simulink model "model"  (R2018b)
settings: Solver=FixedStepAuto  StartTime=0.0  StopTime=sim_time  FixedStep=Ts/10  RelTol=1e-3
StopFcn:
  | %figure;plot(true_position.Data(:,1),true_position.Data(:,2))
values from neighbouring files (symbols this model uses):
  b = 1.115    [main.m]
  bike_params = [g h b a lambda m]    [main.m]
  chalmers = 1    [main.m]
  complementary = 0.985    [main.m]
  D_balancing = 0.0646    [main.m]
  D_heading = 0.01    [main.m]
  D_lateral = 0.01    [main.m]
  g = 9.82    [main.m]
  heading_control = 1    [main.m]
  I_balancing = 1.327    [main.m]
  I_heading = -0.01    [main.m]
  I_lateral = 0    [main.m]
  IMU_height = 0.2    [main.m]
  initial_roll = deg2rad(2)    [main.m]
  initial_rollrate = deg2rad(0)    [main.m]
  initial_steering = deg2rad(0)    [main.m]
  initial_x = 0    [main.m]
  initial_y = 0    [main.m]
  lambda = deg2rad(90-24)    [main.m]
  lateral_control = 0    [main.m]
  mdh = 0    [main.m]
  P_balancing = 3.418    [main.m]
  P_heading = -0.1    [main.m]
  P_lateral = -0.07    [main.m]
  path_tracking = 1    [main.m]
  roll_rate_coef = 0.9    [main.m]
  Ts = 0.01    [main.m]
  v = v_vec(i)    [bike_linear_analysis_balancing.m]    (also in main.m = 3.88888888889)
undefined symbols (not defined in the file or in its folder): A, B, b_compFilter, C, cumulative_dist_along_path, D, IMU_height_model, initial_states, lambda_compFilter, max_roll, min_roll, num_tf_steering, path_x, path_y, Ts_IMU
libraries: simulink x6, dspsigops x2
settings Model: Creator=maximef  LastModifiedBy=maximef

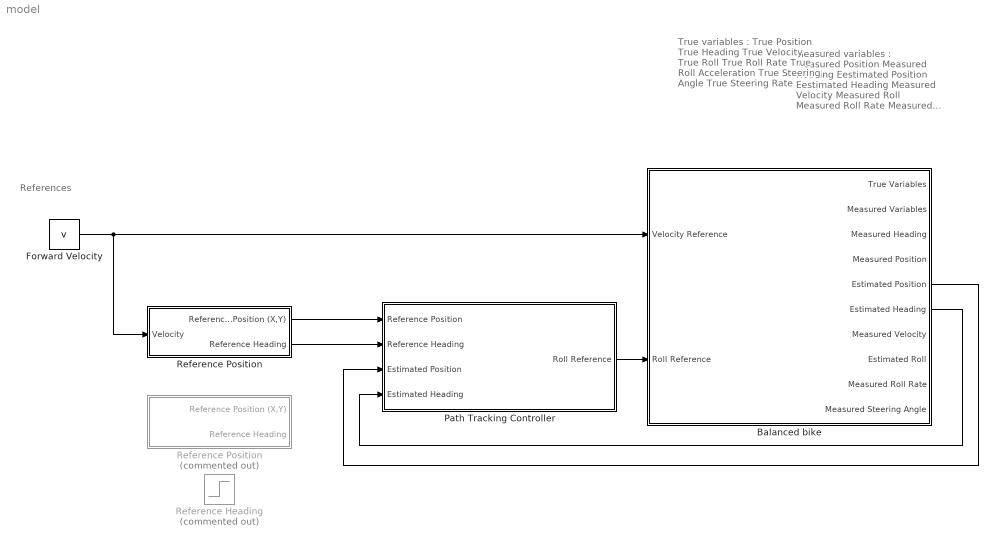
== system model ==
  note: References
  note: Measured variables :
      | Measured Position
      | Measured Heading
      | Eestimated Position
      | Eestimated Heading
      | Measured Velocity
      | Measured Roll
      | Measured Roll Rate
      | Measured Steering Angle
  note: True variables :
      | True Position
      | True Heading
      | True Velocity
      | True Roll
      | True Roll Rate
      | True Roll Acceleration
      | True Steering Angle
      | True Steering Rate
  Balanced bike : Subsystem
  Forward Velocity : Constant  Value=v
  Path Tracking Controller : Subsystem
  Reference Heading : Step  Commented=on  SampleTime=0
  Reference Position : Subsystem  Commented=on
  "Reference Position " : Subsystem
  wires:
  "Reference Position "/1(Reference Position (X,Y)) -> Path Tracking Controller/1(Reference Position)
  "Reference Position "/2(Reference Heading) -> Path Tracking Controller/2(Reference Heading)
  Forward Velocity/1 -> "Reference Position "/1(Velocity), Balanced bike/1(Velocity Reference)
  Path Tracking Controller/1(Roll Reference) -> Balanced bike/2(Roll Reference)
  Balanced bike/5(Estimated Position) -> Path Tracking Controller/3(Estimated Position)
  Balanced bike/6(Estimated Heading) -> Path Tracking Controller/4(Estimated Heading)

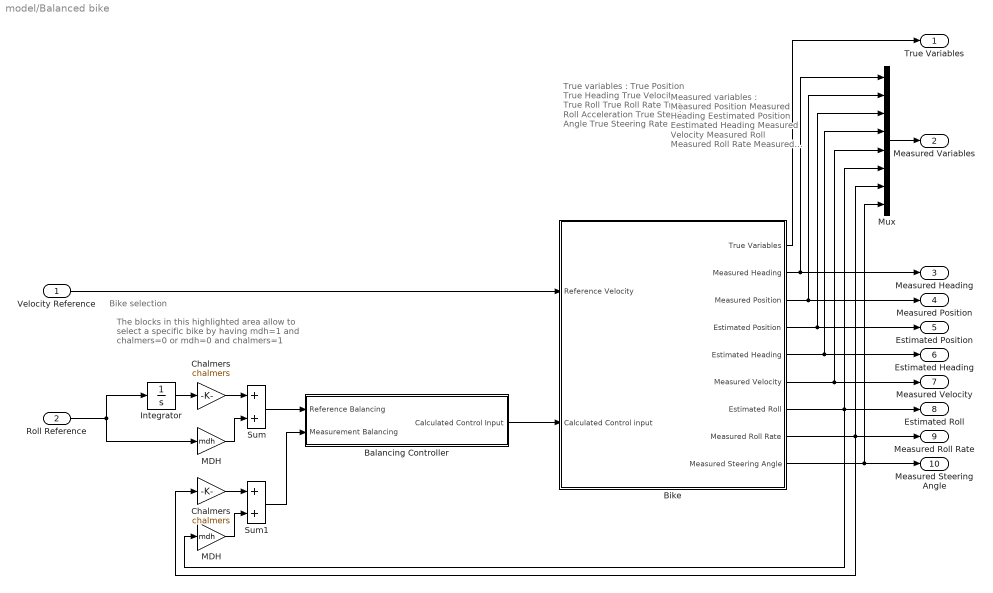
== system model/Balanced bike ==
  note: The blocks in this highlighted area allow
      | to select a specific bike by having
      | mdh=1 and chalmers=0
      | or
      | mdh=0 and chalmers=1
  note: Bike selection
  note: True variables :
      | True Position
      | True Heading
      | True Velocity
      | True Roll
      | True Roll Rate
      | True Roll Acceleration
      | True Steering Angle
      | True Steering Rate
  note: Measured variables :
      | Measured Position
      | Measured Heading
      | Eestimated Position
      | Eestimated Heading
      | Measured Velocity
      | Measured Roll
      | Measured Roll Rate
      | Measured Steering Angle
  Velocity Reference : Inport
  Roll Reference : Inport  Port=2
  Balancing Controller : Subsystem
  Bike : Subsystem
  Chalmers : Gain  Gain=chalmers
  "Chalmers " : Gain  Gain=chalmers
  Integrator : Integrator  InitialCondition=initial_roll
  MDH : Gain  Gain=mdh
  "MDH " : Gain  Gain=mdh
  Mux : Mux  Inputs=8
  Sum : Sum
  Sum1 : Sum
  True Variables : Outport
  Measured Variables : Outport  Port=2
  Measured Heading : Outport  Port=3
  Measured Position : Outport  Port=4
  Estimated Position : Outport  Port=5
  Estimated Heading : Outport  Port=6
  Measured Velocity : Outport  Port=7
  Estimated Roll : Outport  Port=8
  Measured Roll Rate : Outport  Port=9
  Measured Steering Angle : Outport  Port=10
  wires:
  Bike/4(Estimated Position) -> Mux/3, Estimated Position/1
  Bike/3(Measured Position) -> Measured Position/1, Mux/2
  Balancing Controller/1(Calculated Control Input) -> Bike/2(Calculated Control input)
  Velocity Reference/1 -> Bike/1(Reference Velocity)
  Bike/5(Estimated Heading) -> Mux/4, Estimated Heading/1
  Bike/2(Measured Heading) -> Mux/1, Measured Heading/1
  Roll Reference/1 -> Integrator/1, MDH/1
  Chalmers/1 -> Sum/1
  Sum1/1 -> Balancing Controller/2(Measurement Balancing)
  Bike/7(Estimated Roll) -> Mux/6, "MDH "/1, Estimated Roll/1
  Integrator/1 -> Chalmers/1
  Bike/6(Measured Velocity) -> Mux/5, Measured Velocity/1
  Bike/8(Measured Roll Rate) -> Mux/7, "Chalmers "/1, Measured Roll Rate/1
  Bike/9(Measured Steering Angle) -> Mux/8, Measured Steering Angle/1
  "Chalmers "/1 -> Sum1/1
  "MDH "/1 -> Sum1/2
  MDH/1 -> Sum/2
  Sum/1 -> Balancing Controller/1(Reference Balancing)
  Mux/1 -> Measured Variables/1
  Bike/1(True Variables) -> True Variables/1

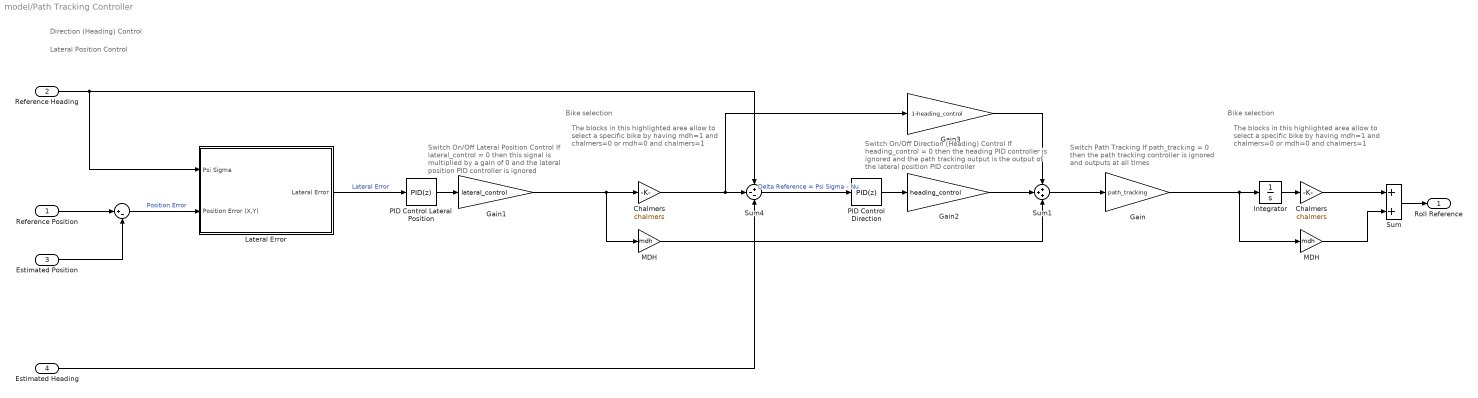
== system model/Path Tracking Controller ==
  note: Direction (Heading) Control
  note: Lateral Position Control
  note: Switch On/Off Lateral Position Control
      | If lateral_control = 0 then this signal
      | is multiplied by a gain of 0 and the
      | lateral position PID controller is ignored
  note: Switch Path Tracking
      | If path_tracking = 0 then the path tracking controller
      | is ignored and outputs at all times
  note: Switch On/Off Direction (Heading) Control
      | If heading_control = 0 then the heading PID controller is ignored
      | and the path tracking output is the output of
      | the lateral position PID controller
  note: Bike selection
  note: The blocks in this highlighted area allow
      | to select a specific bike by having
      | mdh=1 and chalmers=0
      | or
      | mdh=0 and chalmers=1
  note: Bike selection
  note: The blocks in this highlighted area allow
      | to select a specific bike by having
      | mdh=1 and chalmers=0
      | or
      | mdh=0 and chalmers=1
  Reference Position : Inport
  Reference Heading : Inport  Port=2
  Estimated Position : Inport  Port=3
  Estimated Heading : Inport  Port=4
  " " : Sum  Inputs=|+-
  Chalmers : Gain  Gain=chalmers
  "Chalmers " : Gain  Gain=chalmers
  Gain : Gain  Gain=path_tracking
  Gain1 : Gain  Gain=lateral_control
  Gain2 : Gain  Gain=heading_control
  Gain3 : Gain  Gain=1-heading_control
  Integrator : Integrator
  Lateral Error : Subsystem  SystemSampleTime=Ts
  MDH : Gain  Gain=mdh
  "MDH " : Gain  Gain=mdh
  PID Control Lateral Position : simulink/Continuous/PID Controller  Controller=PID  Form=Parallel  TimeDomain=Discrete-time  SampleTime=Ts  IntegratorMethod=Forward Euler  FilterMethod=Forward Euler  ControllerParametersSource=internal  P=P_lateral  I=I_lateral  D=D_lateral  UseFilter=on  N=100  TunerSelectOption=Transfer Function Based (PID Tuner App)  InitialConditionSource=internal  InitialConditionForIntegrator=0  InitialConditionForFilter=0  DifferentiatorICPrevScaledInput=0  ExternalReset=none  TrackingMode=off  Kt=1  LimitOutput=off  UpperSaturationLimit=inf  LowerSaturationLimit=-inf  LinearizeAsGain=on  AntiWindupMode=none  Kb=1  POutMin=[]  POutMax=[]  IOutMin=[]  IOutMax=[]  DOutMin=[]  DOutMax=[]  NOutMin=[]  NOutMax=[]  SumOutMin=[]  SumOutMax=[]  SaturationOutMin=[]  SaturationOutMax=[]  PParamMin=[]  PParamMax=[]  IParamMin=[]  IParamMax=[]  DParamMin=[]  DParamMax=[]  NParamMin=[]  NParamMax=[]  KbParamMin=[]  KbParamMax=[]  KtParamMin=[]  KtParamMax=[]  KbOutMin=[]  KbOutMax=[]  KtOutMin=[]  KtOutMax=[]  IntegratorOutMin=[]  IntegratorOutMax=[]  FilterOutMin=[]  FilterOutMax=[]  SumI1OutMin=[]  SumI1OutMax=[]  SumI2OutMin=[]  SumI2OutMax=[]  SumI3OutMin=[]  SumI3OutMax=[]  SumI4OutMin=[]  SumI4OutMax=[]  SumDOutMin=[]  SumDOutMax=[]  DifferentiatorOutMin=[]  DifferentiatorOutMax=[]  FilterDiffOutCoefMin=[]  FilterDiffOutCoefMax=[]  ReciprocalOutMin=[]  ReciprocalOutMax=[]  SumDenOutMin=[]  SumDenOutMax=[]  SumNumOutMin=[]  SumNumOutMax=[]  DivideOutMin=[]  DivideOutMax=[]  IntegratorContinuousStateAttributes=''  IntegratorStateMustResolveToSignalObject=off  IntegratorRTWStateStorageClass=Auto  FilterContinuousStateAttributes=''  FilterStateMustResolveToSignalObject=off  FilterRTWStateStorageClass=Auto  ParallelPVariant=InternalParameters  IdealPVariant=Disabled  IVariant=InternalParameters  DVariant=InternalParameters  IntegratorVariant=Discrete  SatVariant=Disabled  AWVariant=Passthrough  PCopyVariant=Disabled  TRVariant=Disabled  FdbkBlocksVariant=Forward  IdealPFdbkVariant=Disabled  SatFdbkVariant=Disabled  DerivativeFilterVariant=ForwardEulerFilter  NVariant=InternalParameters  NCopyVariant=Disabled  FilterICVariant=InternalICsFilter  IntegratorICVariant=InternalICs  ExternalResetVariant=Disabled  TRSumVariant=Passthrough  SumFdbkVariant=Disabled  SumVariant=Sum_PID
  PID Control Direction : simulink/Continuous/PID Controller  Controller=PID  Form=Parallel  TimeDomain=Discrete-time  SampleTime=Ts  IntegratorMethod=Forward Euler  FilterMethod=Forward Euler  ControllerParametersSource=internal  P=P_heading  I=I_heading  D=D_heading  UseFilter=on  N=100  TunerSelectOption=Transfer Function Based (PID Tuner App)  InitialConditionSource=internal  InitialConditionForIntegrator=0  InitialConditionForFilter=0  DifferentiatorICPrevScaledInput=0  ExternalReset=none  TrackingMode=off  Kt=1  LimitOutput=off  UpperSaturationLimit=inf  LowerSaturationLimit=-inf  LinearizeAsGain=on  AntiWindupMode=none  Kb=1  POutMin=[]  POutMax=[]  IOutMin=[]  IOutMax=[]  DOutMin=[]  DOutMax=[]  NOutMin=[]  NOutMax=[]  SumOutMin=[]  SumOutMax=[]  SaturationOutMin=[]  SaturationOutMax=[]  PParamMin=[]  PParamMax=[]  IParamMin=[]  IParamMax=[]  DParamMin=[]  DParamMax=[]  NParamMin=[]  NParamMax=[]  KbParamMin=[]  KbParamMax=[]  KtParamMin=[]  KtParamMax=[]  KbOutMin=[]  KbOutMax=[]  KtOutMin=[]  KtOutMax=[]  IntegratorOutMin=[]  IntegratorOutMax=[]  FilterOutMin=[]  FilterOutMax=[]  SumI1OutMin=[]  SumI1OutMax=[]  SumI2OutMin=[]  SumI2OutMax=[]  SumI3OutMin=[]  SumI3OutMax=[]  SumI4OutMin=[]  SumI4OutMax=[]  SumDOutMin=[]  SumDOutMax=[]  DifferentiatorOutMin=[]  DifferentiatorOutMax=[]  FilterDiffOutCoefMin=[]  FilterDiffOutCoefMax=[]  ReciprocalOutMin=[]  ReciprocalOutMax=[]  SumDenOutMin=[]  SumDenOutMax=[]  SumNumOutMin=[]  SumNumOutMax=[]  DivideOutMin=[]  DivideOutMax=[]  IntegratorContinuousStateAttributes=''  IntegratorStateMustResolveToSignalObject=off  IntegratorRTWStateStorageClass=Auto  FilterContinuousStateAttributes=''  FilterStateMustResolveToSignalObject=off  FilterRTWStateStorageClass=Auto  ParallelPVariant=InternalParameters  IdealPVariant=Disabled  IVariant=InternalParameters  DVariant=InternalParameters  IntegratorVariant=Discrete  SatVariant=Disabled  AWVariant=Passthrough  PCopyVariant=Disabled  TRVariant=Disabled  FdbkBlocksVariant=Forward  IdealPFdbkVariant=Disabled  SatFdbkVariant=Disabled  DerivativeFilterVariant=ForwardEulerFilter  NVariant=InternalParameters  NCopyVariant=Disabled  FilterICVariant=InternalICsFilter  IntegratorICVariant=InternalICs  ExternalResetVariant=Disabled  TRSumVariant=Passthrough  SumFdbkVariant=Disabled  SumVariant=Sum_PID
  Sum : Sum
  Sum1 : Sum  Inputs=+++
  Sum4 : Sum  Inputs=+--
  Roll Reference : Outport
  wires:
  Lateral Error/1(Lateral Error) -> PID Control Lateral Position/1  "Lateral Error"
  Estimated Position/1 -> " "/2
  " "/1 -> Lateral Error/2(Position Error (X,Y))  "Position Error"
  Sum4/1 -> PID Control Direction/1  "Delta Reference = Psi Sigma - Nu"
  Estimated Heading/1 -> Sum4/3
  PID Control Lateral Position/1 -> Gain1/1
  Reference Heading/1 -> Lateral Error/1(Psi Sigma), Sum4/1
  Reference Position/1 -> " "/1
  Sum1/1 -> Gain/1
  PID Control Direction/1 -> Gain2/1
  Chalmers/1 -> Gain3/1, Sum4/2
  Gain1/1 -> MDH/1, Chalmers/1
  Gain2/1 -> Sum1/2
  MDH/1 -> Sum1/3
  Gain3/1 -> Sum1/1
  "Chalmers "/1 -> Sum/1
  Gain/1 -> Integrator/1, "MDH "/1
  Integrator/1 -> "Chalmers "/1
  Sum/1 -> Roll Reference/1
  "MDH "/1 -> Sum/2

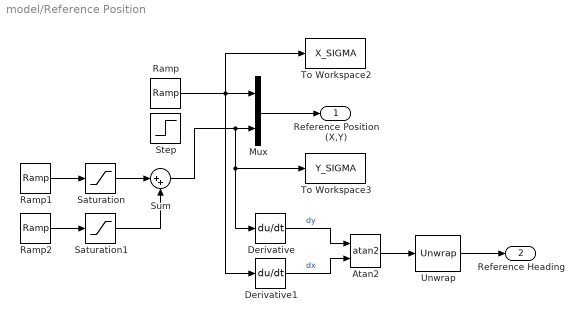
== system model/Reference Position ==
  Atan2 : Trigonometry  Operator=atan2
  Derivative : Derivative
  Derivative1 : Derivative
  Mux : Mux  Inputs=2
  Ramp : simulink/Sources/Ramp  slope=3  start=0  InitialOutput=0
  Ramp1 : simulink/Sources/Ramp  slope=0.01  start=5  InitialOutput=0
  Ramp2 : simulink/Sources/Ramp  slope=-0.01  start=35  InitialOutput=0
  Saturation : Saturate  UpperLimit=0.1  LowerLimit=-0.1
  Saturation1 : Saturate  UpperLimit=0.1  LowerLimit=-0.1
  Step : Step  Time=25  After=0.1  SampleTime=0
  Sum : Sum  Inputs=|++
  To Workspace2 : ToWorkspace  VariableName=X_SIGMA  SaveFormat=Timeseries  SampleTime=Ts
  To Workspace3 : ToWorkspace  VariableName=Y_SIGMA  SaveFormat=Timeseries  SampleTime=Ts
  Unwrap : dspsigops/Unwrap  tol=pi  InputProcessing=Columns as channels (frame based)  running=off
  Reference Position (X,Y) : Outport
  Reference Heading : Outport  Port=2
  wires:
  Mux/1 -> Reference Position (X,Y)/1
  Sum/1 -> Mux/2, Derivative/1, To Workspace3/1
  Ramp/1 -> Mux/1, To Workspace2/1, Derivative1/1
  Derivative1/1 -> Atan2/2  "dx"
  Atan2/1 -> Unwrap/1
  Unwrap/1 -> Reference Heading/1
  Derivative/1 -> Atan2/1  "dy"
  Ramp1/1 -> Saturation/1
  Saturation/1 -> Sum/1
  Saturation1/1 -> Sum/2
  Ramp2/1 -> Saturation1/1

== system model/Reference Position  ==
  Velocity : Inport
  Integrator2 : Integrator
  Mux : Mux  Inputs=2
  Reference Position and Angle Selector : Subsystem
  Reference Position (X,Y) : Outport
  Reference Heading : Outport  Port=2
  wires:
  Reference Position and Angle Selector/3(psi_sigma) -> Reference Heading/1
  Velocity/1 -> Integrator2/1
  Reference Position and Angle Selector/2(Y_sigma) -> Mux/2
  Integrator2/1 -> Reference Position and Angle Selector/1(total travelled distance)  "total travelled distance"
  Reference Position and Angle Selector/1(X_sigma) -> Mux/1
  Mux/1 -> Reference Position (X,Y)/1

== system model/Balanced bike/Balancing Controller ==
  Reference Balancing : Inport
  Measurement Balancing : Inport  Port=2
  Balancing Controller : simulink/Continuous/PID Controller  Controller=PID  Form=Ideal  TimeDomain=Discrete-time  SampleTime=Ts  IntegratorMethod=Trapezoidal  FilterMethod=Forward Euler  ControllerParametersSource=internal  P=P_balancing  I=I_balancing  D=D_balancing  UseFilter=off  N=5  TunerSelectOption=Transfer Function Based (PID Tuner App)  InitialConditionSource=internal  InitialConditionForIntegrator=0  InitialConditionForFilter=0  DifferentiatorICPrevScaledInput=0  ExternalReset=none  TrackingMode=off  Kt=1  LimitOutput=off  UpperSaturationLimit=inf  LowerSaturationLimit=-inf  LinearizeAsGain=on  AntiWindupMode=none  Kb=1  POutMin=[]  POutMax=[]  IOutMin=[]  IOutMax=[]  DOutMin=[]  DOutMax=[]  NOutMin=[]  NOutMax=[]  SumOutMin=[]  SumOutMax=[]  SaturationOutMin=[]  SaturationOutMax=[]  PParamMin=[]  PParamMax=[]  IParamMin=[]  IParamMax=[]  DParamMin=[]  DParamMax=[]  NParamMin=[]  NParamMax=[]  KbParamMin=[]  KbParamMax=[]  KtParamMin=[]  KtParamMax=[]  KbOutMin=[]  KbOutMax=[]  KtOutMin=[]  KtOutMax=[]  IntegratorOutMin=[]  IntegratorOutMax=[]  FilterOutMin=[]  FilterOutMax=[]  SumI1OutMin=[]  SumI1OutMax=[]  SumI2OutMin=[]  SumI2OutMax=[]  SumI3OutMin=[]  SumI3OutMax=[]  SumI4OutMin=[]  SumI4OutMax=[]  SumDOutMin=[]  SumDOutMax=[]  DifferentiatorOutMin=[]  DifferentiatorOutMax=[]  FilterDiffOutCoefMin=[]  FilterDiffOutCoefMax=[]  ReciprocalOutMin=[]  ReciprocalOutMax=[]  SumDenOutMin=[]  SumDenOutMax=[]  SumNumOutMin=[]  SumNumOutMax=[]  DivideOutMin=[]  DivideOutMax=[]  IntegratorContinuousStateAttributes=''  IntegratorStateMustResolveToSignalObject=off  IntegratorRTWStateStorageClass=Auto  FilterContinuousStateAttributes=''  FilterStateMustResolveToSignalObject=off  FilterRTWStateStorageClass=Auto  ParallelPVariant=Passthrough  IdealPVariant=InternalParameters  IVariant=InternalParameters  DVariant=InternalParameters  IntegratorVariant=Discrete  SatVariant=Disabled  AWVariant=Passthrough  PCopyVariant=Disabled  TRVariant=Disabled  FdbkBlocksVariant=Forward  IdealPFdbkVariant=Disabled  SatFdbkVariant=Disabled  DerivativeFilterVariant=Differentiator  NVariant=Passthrough  NCopyVariant=Disabled_SignalSpec  FilterICVariant=InternalICsDifferentiator  IntegratorICVariant=InternalICs  ExternalResetVariant=Disabled  TRSumVariant=Passthrough  SumFdbkVariant=Disabled  SumVariant=Sum_PID
  Sum1 : Sum  Inputs=|+-
  Calculated Control Input : Outport
  wires:
  Reference Balancing/1 -> Sum1/1
  Balancing Controller/1 -> Calculated Control Input/1
  Sum1/1 -> Balancing Controller/1
  Measurement Balancing/1 -> Sum1/2

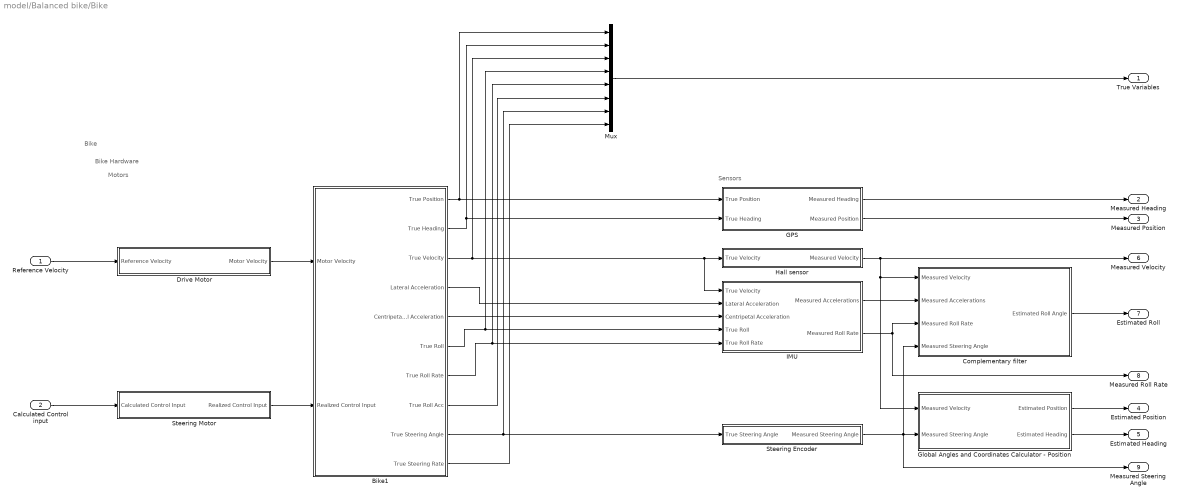
== system model/Balanced bike/Bike ==
  note: Bike
  note: Motors
  note: Bike Hardware
  note: Sensors
  Reference Velocity : Inport
  Calculated Control input : Inport  Port=2
  Bike1 : Subsystem
  Complementary filter : Subsystem  SystemSampleTime=Ts_IMU
  Drive Motor : Subsystem
  GPS : Subsystem  TreatAsAtomicUnit=on
  Global Angles and Coordinates Calculator - Position : Subsystem  SystemSampleTime=Ts
  Hall sensor : Subsystem  TreatAsAtomicUnit=on  SystemSampleTime=Ts
  IMU : Subsystem  TreatAsAtomicUnit=on
  Mux : Mux  Inputs=8
  Steering Encoder : Subsystem  TreatAsAtomicUnit=on  SystemSampleTime=Ts
  Steering Motor : Subsystem
  True Variables : Outport
  Measured Heading : Outport  Port=2
  Measured Position : Outport  Port=3
  Estimated Position : Outport  Port=4
  Estimated Heading : Outport  Port=5
  Measured Velocity : Outport  Port=6
  Estimated Roll : Outport  Port=7
  Measured Roll Rate : Outport  Port=8
  Measured Steering Angle : Outport  Port=9
  wires:
  Global Angles and Coordinates Calculator - Position/1(Estimated Position) -> Estimated Position/1
  Bike1/2(True Heading) -> Mux/2, GPS/2(True Heading)
  Bike1/1(True Position) -> GPS/1(True Position), Mux/1
  Drive Motor/1(Motor Velocity) -> Bike1/1(Motor Velocity)
  Bike1/4(Lateral Acceleration) -> IMU/2(Lateral Acceleration)
  Bike1/9(True Steering Angle) -> Mux/7, Steering Encoder/1(True Steering Angle)
  GPS/2(Measured Position) -> Measured Position/1
  Bike1/6(True Roll) -> Mux/4, IMU/4(True Roll)
  Bike1/3(True Velocity) -> Mux/3, IMU/1(True Velocity), Hall sensor/1(True Velocity)
  Global Angles and Coordinates Calculator - Position/2(Estimated Heading) -> Estimated Heading/1
  Bike1/5(Centripetal Acceleration) -> IMU/3(Centripetal Acceleration)
  Bike1/7(True Roll Rate) -> Mux/5, IMU/5(True Roll Rate)
  GPS/1(Measured Heading) -> Measured Heading/1
  Steering Encoder/1(Measured Steering Angle) -> Measured Steering Angle/1, Global Angles and Coordinates Calculator - Position/2(Measured Steering Angle), Complementary filter/4(Measured Steering Angle)
  IMU/1(Measured Accelerations) -> Complementary filter/2(Measured Accelerations)
  Calculated Control input/1 -> Steering Motor/1(Calculated Control Input)
  Reference Velocity/1 -> Drive Motor/1(Reference Velocity)
  Steering Motor/1(Realized Control Input) -> Bike1/2(Realized Control Input)
  Complementary filter/1(Estimated Roll Angle) -> Estimated Roll/1
  IMU/2(Measured Roll Rate) -> Measured Roll Rate/1, Complementary filter/3(Measured Roll Rate)
  Hall sensor/1(Measured Velocity) -> Measured Velocity/1, Complementary filter/1(Measured Velocity), Global Angles and Coordinates Calculator - Position/1(Measured Velocity)
  Mux/1 -> True Variables/1
  Bike1/8(True Roll Acc) -> Mux/6
  Bike1/10(True Steering Rate) -> Mux/8

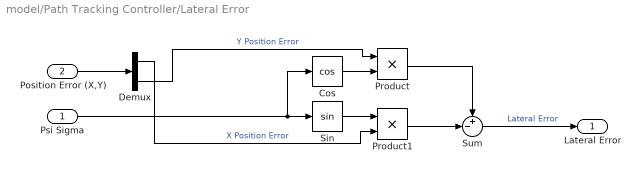
== system model/Path Tracking Controller/Lateral Error ==
  Psi Sigma : Inport
  Position Error (X,Y) : Inport  Port=2
  Cos : Trigonometry  Operator=cos
  Demux : Demux  Outputs=2
  Product : Product
  Product1 : Product
  Sin : Trigonometry
  Sum : Sum  Inputs=+-|
  Lateral Error : Outport
  wires:
  Cos/1 -> Product/2
  Sin/1 -> Product1/1
  Psi Sigma/1 -> Cos/1, Sin/1
  Product1/1 -> Sum/2
  Product/1 -> Sum/1
  Sum/1 -> Lateral Error/1  "Lateral Error"
  Demux/1 -> Product1/2  "X Position Error"
  Demux/2 -> Product/1  "Y Position Error"
  Position Error (X,Y)/1 -> Demux/1

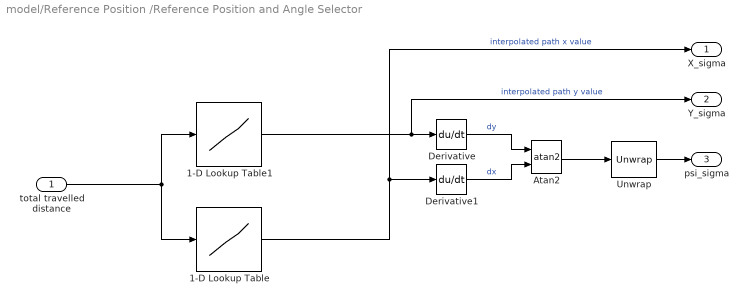
== system model/Reference Position /Reference Position and Angle Selector ==
  total travelled distance : Inport
  1-D Lookup Table : Lookup_n-D  NumberOfTableDimensions=1  BreakpointsForDimension1=cumulative_dist_along_path  Table=path_x  ExtrapMethod=Clip  DiagnosticForOutOfRangeInput=Error  InternalRulePriority=Speed  RndMeth=Simplest  InputSameDT=on
  1-D Lookup Table1 : Lookup_n-D  NumberOfTableDimensions=1  BreakpointsForDimension1=cumulative_dist_along_path  Table=path_y  ExtrapMethod=Clip  DiagnosticForOutOfRangeInput=Error  InternalRulePriority=Speed  RndMeth=Simplest  InputSameDT=on
  Atan2 : Trigonometry  Operator=atan2
  Derivative : Derivative
  Derivative1 : Derivative
  Unwrap : dspsigops/Unwrap  tol=pi  InputProcessing=Columns as channels (frame based)  running=off
  X_sigma : Outport
  Y_sigma : Outport  Port=2
  psi_sigma : Outport  Port=3
  wires:
  total travelled distance/1 -> 1-D Lookup Table1/1, 1-D Lookup Table/1
  Unwrap/1 -> psi_sigma/1
  1-D Lookup Table/1 -> X_sigma/1, Derivative1/1  "interpolated path x value"
  Derivative1/1 -> Atan2/2  "dx"
  Derivative/1 -> Atan2/1  "dy"
  Atan2/1 -> Unwrap/1
  1-D Lookup Table1/1 -> Y_sigma/1, Derivative/1  "interpolated path y value"

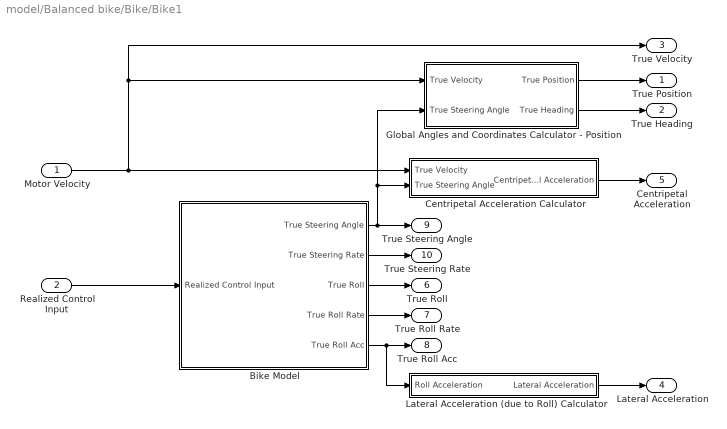
== system model/Balanced bike/Bike/Bike1 ==
  Motor Velocity : Inport
  Realized Control Input : Inport  Port=2
  Bike Model : Subsystem
  Centripetal Acceleration Calculator : Subsystem
  Global Angles and Coordinates Calculator - Position : Subsystem  SystemSampleTime=Ts
  Lateral Acceleration (due to Roll) Calculator : Subsystem
  True Position : Outport
  True Heading : Outport  Port=2
  True Velocity : Outport  Port=3
  Lateral Acceleration : Outport  Port=4
  Centripetal Acceleration : Outport  Port=5
  True Roll : Outport  Port=6
  True Roll Rate : Outport  Port=7
  True Roll Acc : Outport  Port=8
  True Steering Angle : Outport  Port=9
  True Steering Rate : Outport  Port=10
  wires:
  Global Angles and Coordinates Calculator - Position/1(True Position) -> True Position/1
  Global Angles and Coordinates Calculator - Position/2(True Heading) -> True Heading/1
  Motor Velocity/1 -> Centripetal Acceleration Calculator/1(True Velocity), True Velocity/1, Global Angles and Coordinates Calculator - Position/1(True Velocity)
  Realized Control Input/1 -> Bike Model/1(Realized Control Input)
  Bike Model/3(True Roll) -> True Roll/1
  Lateral Acceleration (due to Roll) Calculator/1(Lateral Acceleration) -> Lateral Acceleration/1
  Centripetal Acceleration Calculator/1(Centripetal Acceleration) -> Centripetal Acceleration/1
  Bike Model/4(True Roll Rate) -> True Roll Rate/1
  Bike Model/5(True Roll Acc) -> Lateral Acceleration (due to Roll) Calculator/1(Roll Acceleration), True Roll Acc/1
  Bike Model/1(True Steering Angle) -> True Steering Angle/1, Global Angles and Coordinates Calculator - Position/2(True Steering Angle), Centripetal Acceleration Calculator/2(True Steering Angle)
  Bike Model/2(True Steering Rate) -> True Steering Rate/1

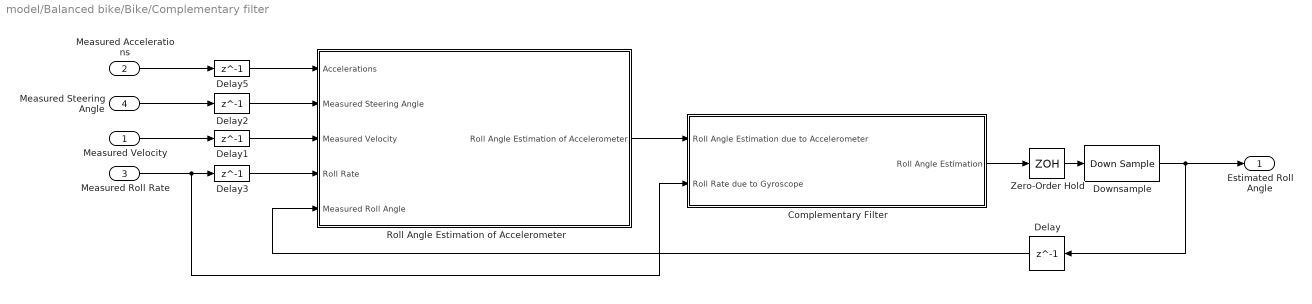
== system model/Balanced bike/Bike/Complementary filter ==
  Measured Velocity : Inport
  Measured Accelerations : Inport  Port=2
  Measured Roll Rate : Inport  Port=3
  Measured Steering Angle : Inport  Port=4
  Complementary Filter : Subsystem  TreatAsAtomicUnit=on  SystemSampleTime=Ts_IMU
  Delay{,1..3,5} (5 alike) : Delay  DelayLength=1
  Downsample : DownSample  N=Ts/Ts_IMU  RateOptions=Allow multirate processing
  Roll Angle Estimation of Accelerometer : Subsystem
  Zero-Order Hold : ZeroOrderHold  SampleTime=Ts_IMU
  Estimated Roll Angle : Outport
  wires:
  Roll Angle Estimation of Accelerometer/1(Roll Angle Estimation of Accelerometer) -> Complementary Filter/1(Roll Angle Estimation due to Accelerometer)
  Measured Roll Rate/1 -> Delay3/1, Complementary Filter/2(Roll Rate due to Gyroscope)
  Zero-Order Hold/1 -> Downsample/1
  Measured Accelerations/1 -> Delay5/1
  Measured Steering Angle/1 -> Delay2/1
  Measured Velocity/1 -> Delay1/1
  Delay/1 -> Roll Angle Estimation of Accelerometer/5(Measured Roll Angle)
  Delay1/1 -> Roll Angle Estimation of Accelerometer/3(Measured Velocity)
  Delay2/1 -> Roll Angle Estimation of Accelerometer/2(Measured Steering Angle)
  Delay5/1 -> Roll Angle Estimation of Accelerometer/1(Accelerations)
  Complementary Filter/1(Roll Angle Estimation) -> Zero-Order Hold/1
  Downsample/1 -> Estimated Roll Angle/1, Delay/1
  Delay3/1 -> Roll Angle Estimation of Accelerometer/4(Roll Rate)

== system model/Balanced bike/Bike/Drive Motor ==
  Reference Velocity : Inport
  Motor Velocity : Outport
  wires:
  Reference Velocity/1 -> Motor Velocity/1

== system model/Balanced bike/Bike/GPS ==
  True Position : Inport
  True Heading : Inport  Port=2
  GPS Heading : ZeroOrderHold  SampleTime=-1
  GPS Position : ZeroOrderHold  SampleTime=-1
  Measured Heading : Outport
  Measured Position : Outport  Port=2
  wires:
  True Position/1 -> GPS Position/1
  True Heading/1 -> GPS Heading/1
  GPS Heading/1 -> Measured Heading/1
  GPS Position/1 -> Measured Position/1

== system model/Balanced bike/Bike/Global Angles and Coordinates Calculator - Position ==
  Measured Velocity : Inport
  Measured Steering Angle : Inport  Port=2
  Gain1 : Gain  Gain=sin(lambda)
  Measured Bike Angles to Global Angles : Subsystem
  Measured Global Angles to Global Coordinates : Subsystem
  Sum : Sum  Inputs=++|
  Estimated Position : Outport
  Estimated Heading : Outport  Port=2
  wires:
  Measured Bike Angles to Global Angles/1(Psi) -> Sum/2, Measured Global Angles to Global Coordinates/2(Psi)
  Gain1/1 -> Measured Bike Angles to Global Angles/2(Measured Steering Angle)
  Sum/1 -> Estimated Heading/1
  Measured Bike Angles to Global Angles/2(Beta) -> Sum/1, Measured Global Angles to Global Coordinates/3(Beta)
  Measured Global Angles to Global Coordinates/1("Position (X, Y)") -> Estimated Position/1
  Measured Velocity/1 -> Measured Global Angles to Global Coordinates/1(Velocity), Measured Bike Angles to Global Angles/1(Velocity)
  Measured Steering Angle/1 -> Gain1/1

== system model/Balanced bike/Bike/Hall sensor ==
  True Velocity : Inport
  Zero-Order Hold : ZeroOrderHold  SampleTime=Ts
  Measured Velocity : Outport
  wires:
  True Velocity/1 -> Zero-Order Hold/1
  Zero-Order Hold/1 -> Measured Velocity/1

== system model/Balanced bike/Bike/IMU ==
  True Velocity : Inport
  Lateral Acceleration : Inport  Port=2
  Centripetal Acceleration : Inport  Port=3
  True Roll : Inport  Port=4
  True Roll Rate : Inport  Port=5
  IMU Accelerometer : Subsystem
  IMU Gyroscope : ZeroOrderHold  SampleTime=-1
  Measured Accelerations : Outport
  Measured Roll Rate : Outport  Port=2
  wires:
  True Velocity/1 -> IMU Accelerometer/3(True Velocity)
  Lateral Acceleration/1 -> IMU Accelerometer/1(Lateral Acceleration of the IMU due to Roll)
  Centripetal Acceleration/1 -> IMU Accelerometer/2(Centripetal Acceleration due to Path Curvature)
  True Roll/1 -> IMU Accelerometer/4(True Roll Angle)
  IMU Accelerometer/1(Accelerations) -> Measured Accelerations/1
  IMU Gyroscope/1 -> Measured Roll Rate/1
  True Roll Rate/1 -> IMU Gyroscope/1

== system model/Balanced bike/Bike/Steering Encoder ==
  True Steering Angle : Inport
  Zero-Order Hold : ZeroOrderHold  SampleTime=Ts
  Measured Steering Angle : Outport
  wires:
  True Steering Angle/1 -> Zero-Order Hold/1
  Zero-Order Hold/1 -> Measured Steering Angle/1

== system model/Balanced bike/Bike/Steering Motor ==
  Calculated Control Input : Inport
  Steering motor transfer function Steering Rate Reference to Realized Steering Rate : TransferFcn  Numerator=[num_tf_steering]  Denominator=[den_tf_steering(1:end-1)]
  Realized Control Input : Outport
  wires:
  Steering motor transfer function Steering Rate Reference to Realized Steering Rate/1 -> Realized Control Input/1
  Calculated Control Input/1 -> Steering motor transfer function Steering Rate Reference to Realized Steering Rate/1

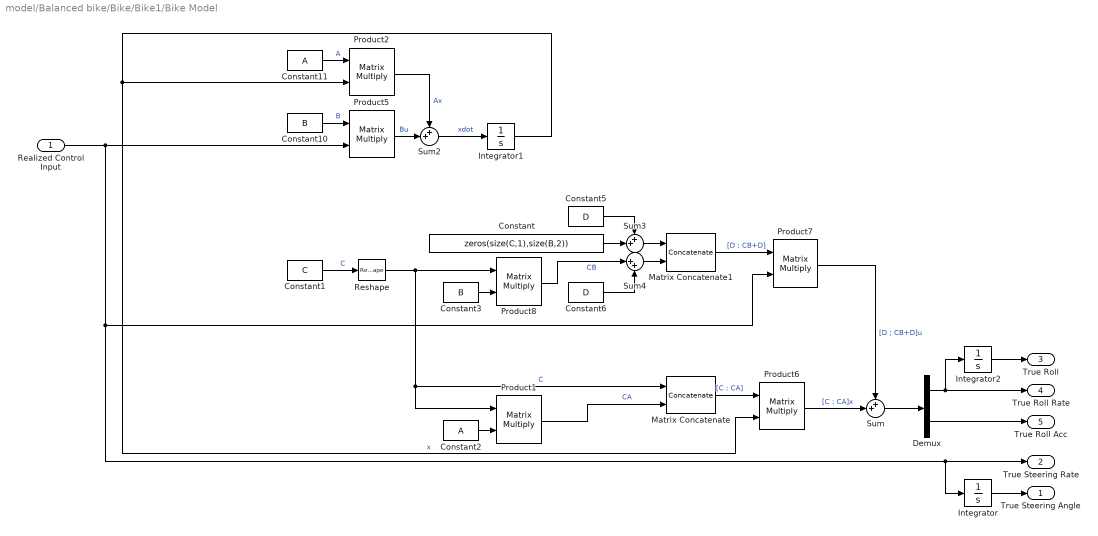
== system model/Balanced bike/Bike/Bike1/Bike Model ==
  Realized Control Input : Inport
  Constant : Constant  Value=zeros(size(C,1),size(B,2))
  Constant1 : Constant  Value=C
  Constant10 : Constant  Value=B
  Constant11 : Constant  Value=A
  Constant2 : Constant  Value=A
  Constant3 : Constant  Value=B
  Constant5 : Constant  Value=D
  Constant6 : Constant  Value=D
  Demux : Demux  Outputs=2
  Integrator : Integrator  InitialCondition=initial_steering
  Integrator1 : Integrator  InitialCondition=[C ; C*A]\[initial_roll ; initial_rollrate]
  Integrator2 : Integrator  InitialCondition=initial_roll
  Matrix Concatenate : Concatenate  Mode=Multidimensional array
  Matrix Concatenate1 : Concatenate  Mode=Multidimensional array
  Product{1..2,5..8} (6 alike) : Product  SCDEnableBlockLinearizationSpecification=on  Multiplication=Matrix(*)
  Reshape : Reshape  OutputDimensionality=Customize  OutputDimensions=[size(C,1),size(C,2)]
  Sum : Sum  Inputs=++|
  Sum2 : Sum  Inputs=++|
  Sum3 : Sum  Inputs=++|
  Sum4 : Sum  Inputs=|++
  True Steering Angle : Outport
  True Steering Rate : Outport  Port=2
  True Roll : Outport  Port=3
  True Roll Rate : Outport  Port=4
  True Roll Acc : Outport  Port=5
  wires:
  Reshape/1 -> Product1/1, Matrix Concatenate/1, Product8/1  "C"
  Sum/1 -> Demux/1
  Constant1/1 -> Reshape/1  "C"
  Matrix Concatenate/1 -> Product6/1  "[C ; CA]"
  Product5/1 -> Sum2/2  "Bu"
  Matrix Concatenate1/1 -> Product7/1  "[D ; CB+D]"
  Constant11/1 -> Product2/1  "A"
  Constant3/1 -> Product8/2
  Product6/1 -> Sum/2  "[C ; CA]x"
  Sum2/1 -> Integrator1/1  "xdot"
  Product2/1 -> Sum2/1  "Ax"
  Product1/1 -> Matrix Concatenate/2  "CA"
  Product8/1 -> Sum4/1  "CB"
  Integrator1/1 -> Product2/2, Product6/2  "x"
  Constant2/1 -> Product1/2
  Product7/1 -> Sum/1  "[D ; CB+D]u"
  Constant10/1 -> Product5/1  "B"
  Realized Control Input/1 -> Product7/2, True Steering Rate/1, Integrator/1, Product5/2
  Sum3/1 -> Matrix Concatenate1/1
  Constant/1 -> Sum3/2
  Constant5/1 -> Sum3/1
  Sum4/1 -> Matrix Concatenate1/2
  Constant6/1 -> Sum4/2
  Integrator/1 -> True Steering Angle/1
  Demux/2 -> True Roll Acc/1
  Demux/1 -> True Roll Rate/1, Integrator2/1
  Integrator2/1 -> True Roll/1

== system model/Balanced bike/Bike/Bike1/Centripetal Acceleration Calculator ==
  True Velocity : Inport
  True Steering Angle : Inport  Port=2
  Divide : Product  Inputs=*/
  Gain : Gain  Gain=sin(lambda)
  Multiply : Product
  Square : Math  Operator=square  SaturateOnIntegerOverflow=on
  Tan : Trigonometry  Operator=tan
  b Real Bike : Constant  Value=b
  Centripetal Acceleration : Outport
  wires:
  True Velocity/1 -> Square/1
  Square/1 -> Divide/1
  b Real Bike/1 -> Divide/2
  True Steering Angle/1 -> Gain/1
  Divide/1 -> Multiply/1
  Tan/1 -> Multiply/2
  Multiply/1 -> Centripetal Acceleration/1
  Gain/1 -> Tan/1

== system model/Balanced bike/Bike/Bike1/Global Angles and Coordinates Calculator - Position ==
  note: True Steering
      | Angle
  True Velocity : Inport
  True Steering Angle : Inport  Port=2
  Gain1 : Gain  Gain=sin(lambda)
  Measured Bike Angles to Global Angles : Subsystem
  Measured Global Angles to Global Coordinates : Subsystem
  Sum : Sum  Inputs=++|
  True Position : Outport
  True Heading : Outport  Port=2
  wires:
  Measured Bike Angles to Global Angles/1(Psi) -> Sum/2, Measured Global Angles to Global Coordinates/2(Psi)
  Gain1/1 -> Measured Bike Angles to Global Angles/2(Measured Steering Angle)
  Sum/1 -> True Heading/1
  Measured Bike Angles to Global Angles/2(Beta) -> Sum/1, Measured Global Angles to Global Coordinates/3(Beta)
  Measured Global Angles to Global Coordinates/1("Position (X, Y)") -> True Position/1
  True Velocity/1 -> Measured Global Angles to Global Coordinates/1(Velocity), Measured Bike Angles to Global Angles/1(Velocity)
  True Steering Angle/1 -> Gain1/1

== system model/Balanced bike/Bike/Bike1/Lateral Acceleration (due to Roll) Calculator ==
  Roll Acceleration : Inport
  Constant3 : Constant  Value=IMU_height
  Multiply : Product
  Lateral Acceleration : Outport
  wires:
  Multiply/1 -> Lateral Acceleration/1
  Constant3/1 -> Multiply/1
  Roll Acceleration/1 -> Multiply/2

== system model/Balanced bike/Bike/Complementary filter/Complementary Filter ==
  Roll Angle Estimation due to Accelerometer : Inport
  Roll Rate due to Gyroscope : Inport  Port=2
  Delay : Delay  DelayLength=1  InitialCondition=initial_states(1)
  Gain2 : Gain  Gain=complementary
  Gain3 : Gain  Gain=1-complementary
  Gain4 : Gain  Gain=Ts_IMU
  Sum3 : Sum  Inputs=|++
  Sum4 : Sum  Inputs=++|
  Roll Angle Estimation : Outport
  wires:
  Roll Angle Estimation due to Accelerometer/1 -> Gain3/1  "Roll_acc"
  Sum3/1 -> Gain2/1
  Roll Rate due to Gyroscope/1 -> Gain4/1
  Delay/1 -> Sum3/2
  Gain4/1 -> Sum3/1
  Gain2/1 -> Sum4/2
  Gain3/1 -> Sum4/1
  Sum4/1 -> Delay/1, Roll Angle Estimation/1

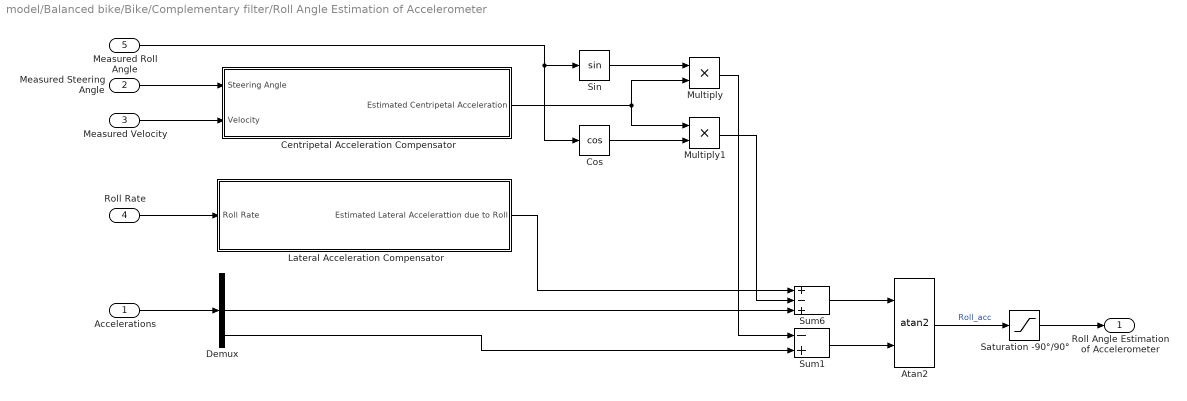
== system model/Balanced bike/Bike/Complementary filter/Roll Angle Estimation of Accelerometer ==
  Accelerations : Inport
  Measured Steering Angle : Inport  Port=2
  Measured Velocity : Inport  Port=3
  Roll Rate : Inport  Port=4
  Measured Roll Angle : Inport  Port=5
  Atan2 : Trigonometry  Operator=atan2
  Centripetal Acceleration Compensator : Subsystem
  Cos : Trigonometry  Operator=cos
  Demux : Demux  Outputs=3
  Lateral Acceleration Compensator : Subsystem
  Multiply : Product
  Multiply1 : Product
  Saturation -90°/90° : Saturate  UpperLimit=max_roll  LowerLimit=min_roll
  Sin : Trigonometry
  Sum1 : Sum  Inputs=-+
  Sum6 : Sum  Inputs=+-+
  Roll Angle Estimation of Accelerometer : Outport
  wires:
  Sum1/1 -> Atan2/2
  Lateral Acceleration Compensator/1(Estimated Lateral Accelerattion due to Roll) -> Sum6/1
  Atan2/1 -> Saturation -90°/90°/1  "Roll_acc"
  Roll Rate/1 -> Lateral Acceleration Compensator/1(Roll Rate)
  Accelerations/1 -> Demux/1
  Measured Velocity/1 -> Centripetal Acceleration Compensator/2(Velocity)
  Centripetal Acceleration Compensator/1(Estimated Centripetal Acceleration) -> Multiply/2, Multiply1/1
  Measured Roll Angle/1 -> Sin/1, Cos/1
  Cos/1 -> Multiply1/2
  Sin/1 -> Multiply/1
  Multiply1/1 -> Sum6/2
  Demux/3 -> Sum1/2
  Multiply/1 -> Sum1/1
  Sum6/1 -> Atan2/1
  Measured Steering Angle/1 -> Centripetal Acceleration Compensator/1(Steering Angle)
  Demux/2 -> Sum6/3
  Saturation -90°/90°/1 -> Roll Angle Estimation of Accelerometer/1

== system model/Balanced bike/Bike/Global Angles and Coordinates Calculator - Position/Measured Bike Angles to Global Angles ==
  Velocity : Inport
  Measured Steering Angle : Inport  Port=2
  " Bike Parameters Model " : Constant  Value=bike_params
  Integrator : Integrator
  MATLAB Function : MATLAB Function  TreatAsAtomicUnit=on
  Psi : Outport
  Beta : Outport  Port=2
  wires:
  MATLAB Function/2(beta) -> Beta/1
  MATLAB Function/1(psi_d) -> Integrator/1
  Integrator/1 -> Psi/1
  " Bike Parameters Model "/1 -> MATLAB Function/2(parameters_model)
  Measured Steering Angle/1 -> MATLAB Function/3(delta)
  Velocity/1 -> MATLAB Function/1(v)

== system model/Balanced bike/Bike/Global Angles and Coordinates Calculator - Position/Measured Global Angles to Global Coordinates ==
  Velocity : Inport
  Psi : Inport  Port=2
  Beta : Inport  Port=3
  Integrator1 : Integrator  InitialCondition=initial_x
  Integrator2 : Integrator  InitialCondition=initial_y
  MATLAB Function1 : MATLAB Function  TreatAsAtomicUnit=on
  Mux : Mux  Inputs=2
  "Position (X, Y)" : Outport
  wires:
  MATLAB Function1/2(Ydot) -> Integrator2/1  "Ydot"
  MATLAB Function1/1(Xdot) -> Integrator1/1  "Xdot"
  Psi/1 -> MATLAB Function1/2(psi)
  Beta/1 -> MATLAB Function1/3(beta)
  Velocity/1 -> MATLAB Function1/1(v)
  Integrator2/1 -> Mux/2
  Integrator1/1 -> Mux/1
  Mux/1 -> "Position (X, Y)"/1

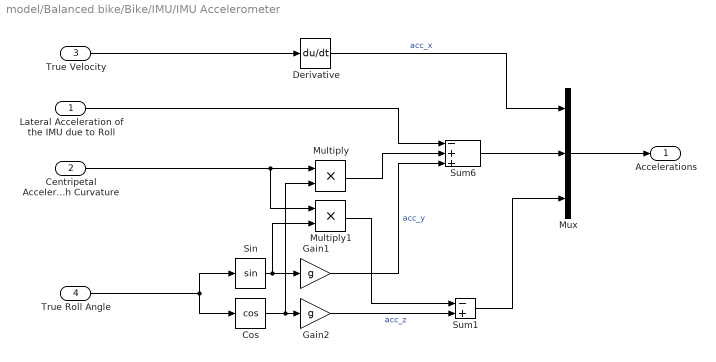
== system model/Balanced bike/Bike/IMU/IMU Accelerometer ==
  Lateral Acceleration of the IMU due to Roll : Inport
  Centripetal Acceleration due to Path Curvature : Inport  Port=2
  True Velocity : Inport  Port=3
  True Roll Angle : Inport  Port=4
  Cos : Trigonometry  Operator=cos
  Derivative : Derivative  CoefficientInTFapproximation=-1
  Gain1 : Gain  Gain=g
  Gain2 : Gain  Gain=g
  Multiply : Product
  Multiply1 : Product
  Mux : Mux  Inputs=3
  Sin : Trigonometry
  Sum1 : Sum  Inputs=-+
  Sum6 : Sum  Inputs=-++
  Accelerations : Outport
  wires:
  Multiply/1 -> Sum6/2
  Gain1/1 -> Sum6/3  "acc_y"
  Sin/1 -> Multiply1/2, Gain1/1
  Derivative/1 -> Mux/1  "acc_x"
  Cos/1 -> Multiply/2, Gain2/1
  Gain2/1 -> Sum1/2  "acc_z"
  True Roll Angle/1 -> Sin/1, Cos/1
  True Velocity/1 -> Derivative/1
  Centripetal Acceleration due to Path Curvature/1 -> Multiply1/1, Multiply/1
  Multiply1/1 -> Sum1/1
  Sum1/1 -> Mux/3
  Mux/1 -> Accelerations/1
  Sum6/1 -> Mux/2
  Lateral Acceleration of the IMU due to Roll/1 -> Sum6/1

== system model/Balanced bike/Bike/Bike1/Global Angles and Coordinates Calculator - Position/Measured Bike Angles to Global Angles ==
  Velocity : Inport
  Measured Steering Angle : Inport  Port=2
  " Bike Parameters Model " : Constant  Value=bike_params
  Integrator : Integrator
  MATLAB Function : MATLAB Function  TreatAsAtomicUnit=on
  Psi : Outport
  Beta : Outport  Port=2
  wires:
  MATLAB Function/2(beta) -> Beta/1
  MATLAB Function/1(psi_d) -> Integrator/1
  Integrator/1 -> Psi/1
  " Bike Parameters Model "/1 -> MATLAB Function/2(bike_params)
  Measured Steering Angle/1 -> MATLAB Function/3(delta)
  Velocity/1 -> MATLAB Function/1(v)

== system model/Balanced bike/Bike/Bike1/Global Angles and Coordinates Calculator - Position/Measured Global Angles to Global Coordinates ==
  Velocity : Inport
  Psi : Inport  Port=2
  Beta : Inport  Port=3
  Integrator1 : Integrator
  Integrator2 : Integrator
  MATLAB Function1 : MATLAB Function  TreatAsAtomicUnit=on
  Mux : Mux  Inputs=2
  "Position (X, Y)" : Outport
  wires:
  MATLAB Function1/2(Ydot) -> Integrator2/1  "Ydot"
  MATLAB Function1/1(Xdot) -> Integrator1/1  "Xdot"
  Psi/1 -> MATLAB Function1/2(psi)
  Beta/1 -> MATLAB Function1/3(beta)
  Velocity/1 -> MATLAB Function1/1(v)
  Integrator2/1 -> Mux/2
  Integrator1/1 -> Mux/1
  Mux/1 -> "Position (X, Y)"/1

== system model/Balanced bike/Bike/Complementary filter/Roll Angle Estimation of Accelerometer/Centripetal Acceleration Compensator ==
  Steering Angle : Inport
  Velocity : Inport  Port=2
  Bike Model b : Constant  Value=b_compFilter
  Divide : Product  Inputs=*/
  Gain : Gain  Gain=sin(lambda_compFilter)
  Multiply : Product
  Square : Math  Operator=square  SaturateOnIntegerOverflow=on
  Tan : Trigonometry  Operator=tan
  Estimated Centripetal Acceleration : Outport
  wires:
  Velocity/1 -> Square/1
  Square/1 -> Divide/1
  Bike Model b/1 -> Divide/2
  Steering Angle/1 -> Gain/1
  Divide/1 -> Multiply/1
  Tan/1 -> Multiply/2
  Multiply/1 -> Estimated Centripetal Acceleration/1
  Gain/1 -> Tan/1

== system model/Balanced bike/Bike/Complementary filter/Roll Angle Estimation of Accelerometer/Lateral Acceleration Compensator ==
  Roll Rate : Inport
  Constant4 : Constant  Value=IMU_height_model
  Low Pass Filter : Subsystem
  Multiply1 : Product
  Numerical Derivative : Subsystem
  Estimated Lateral Accelerattion due to Roll : Outport
  wires:
  Numerical Derivative/1(Roll Acceleration) -> Multiply1/2  "roll angular acceleration"
  Roll Rate/1 -> Low Pass Filter/1(Roll Rate)
  Constant4/1 -> Multiply1/1
  Multiply1/1 -> Estimated Lateral Accelerattion due to Roll/1  "lateral acceleration"
  Low Pass Filter/1(Filtered Roll Rate) -> Numerical Derivative/1(Roll Rate)

== system model/Balanced bike/Bike/Complementary filter/Roll Angle Estimation of Accelerometer/Lateral Acceleration Compensator/Low Pass Filter ==
  Roll Rate : Inport
  Delay18 : Delay  DelayLength=1
  Gain4 : Gain  Gain=roll_rate_coef
  Gain6 : Gain  Gain=1-roll_rate_coef
  Scope7 : Scope  NumInputPorts=2
  Sum4 : Sum  Inputs=|++
  Filtered Roll Rate : Outport
  wires:
  Gain6/1 -> Sum4/1
  Gain4/1 -> Sum4/2
  Sum4/1 -> Filtered Roll Rate/1, Delay18/1, Scope7/2  "Filtered Roll Rate"
  Delay18/1 -> Gain4/1
  Roll Rate/1 -> Scope7/1, Gain6/1  "Measured Roll Rate"

== system model/Balanced bike/Bike/Complementary filter/Roll Angle Estimation of Accelerometer/Lateral Acceleration Compensator/Numerical Derivative ==
  Roll Rate : Inport
  Delay18 : Delay  DelayLength=1
  Gain3 : Gain  Gain=1/Ts_IMU
  Sum3 : Sum  Inputs=|+-
  Roll Acceleration : Outport
  wires:
  Sum3/1 -> Gain3/1
  Delay18/1 -> Sum3/2
  Roll Rate/1 -> Sum3/1, Delay18/1
  Gain3/1 -> Roll Acceleration/1

== matlab function model/Balanced bike/Bike/Global Angles and Coordinates Calculator - Position/Measured Bike Angles to Global Angles/MATLAB Function ==
  data: v input; parameters_model input; delta input; psi_d output; beta output
function [psi_d, beta]  = fcn(v, parameters_model, delta)

b = parameters_model(3);
a = parameters_model(4);

beta = atan((a / (b)) * tan(delta));
psi_d = (v / a) * sin(beta);

== matlab function model/Balanced bike/Bike/Global Angles and Coordinates Calculator - Position/Measured Global Angles to Global Coordinates/MATLAB Function1 ==
  data: v input; psi input; Xdot output; beta input; Ydot output
function [Xdot, Ydot]  = fcn(v, psi, beta)

Xdot = v * cos(psi + beta);
Ydot = v * sin(psi + beta);

== matlab function model/Balanced bike/Bike/Bike1/Global Angles and Coordinates Calculator - Position/Measured Bike Angles to Global Angles/MATLAB Function ==
  data: v input; bike_params input; delta input; psi_d output; beta output
function [psi_d, beta]  = fcn(v, bike_params, delta)

b = bike_params(3);
a = bike_params(4);

beta = atan((a / (b)) * tan(delta));
psi_d = (v / a) * sin(beta);

== matlab function model/Balanced bike/Bike/Bike1/Global Angles and Coordinates Calculator - Position/Measured Global Angles to Global Coordinates/MATLAB Function1 ==
  data: v input; psi input; Xdot output; beta input; Ydot output
function [Xdot, Ydot]  = fcn(v, psi, beta)

Xdot = v * cos(psi + beta);
Ydot = v * sin(psi + beta);
